simulink model "opt_qvm_bocsh_contr"  (Simulink 4.0)
settings: Solver=ode45  StartTime=0.0  StopTime=10.0  RelTol=1e-3
libraries: simulink_extras x7
settings Model: LastModifiedBy=krangelo  BooleanDataType=on

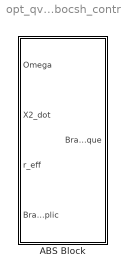
== system opt_qvm_bocsh_contr ==
  ABS Block : Subsystem  SimViewingDevice=off  mask{R1=19000, R2=19000, Bmax=1300, TO=0.006, TC=0.050, Slip=18, Slipmin=17, neg_a=60, pos_a=3, A=10, om_dot_om=3}
      mask prompts: R1 "R1 - Rate of incerase of the  Breake Torque. [Nm/s]"; R2 "R2 - Rate of decerase of the  Breake Torque. [Nm/s]"; Bmax "Bmax - Max. Value of the Brake Torque. [Nm]"; TO "TO - Inlet Valve open time [s]"; TC "TC - Inlet Valve close time [s]"; Slip "Desired slip [%]"; Slipmin "Slipmin - Minimum slip level"; neg_a "-a - Threshold value of the wheel peripheral deceleration [m/s^2]"; pos_a "+a - Threshold value of the wheel peripheral acceleration [m/s^2]"; A "A - Threshold value of the wheel peripheral acceleration [m/s^2]"; om_dot_om "Omdot/Omega -Threshold value of the ratio Om_dot / Om [Hz]"
      settings: Permissions=ReadWrite  RTWFcnNameOpts=Auto  RTWFileNameOpts=Auto

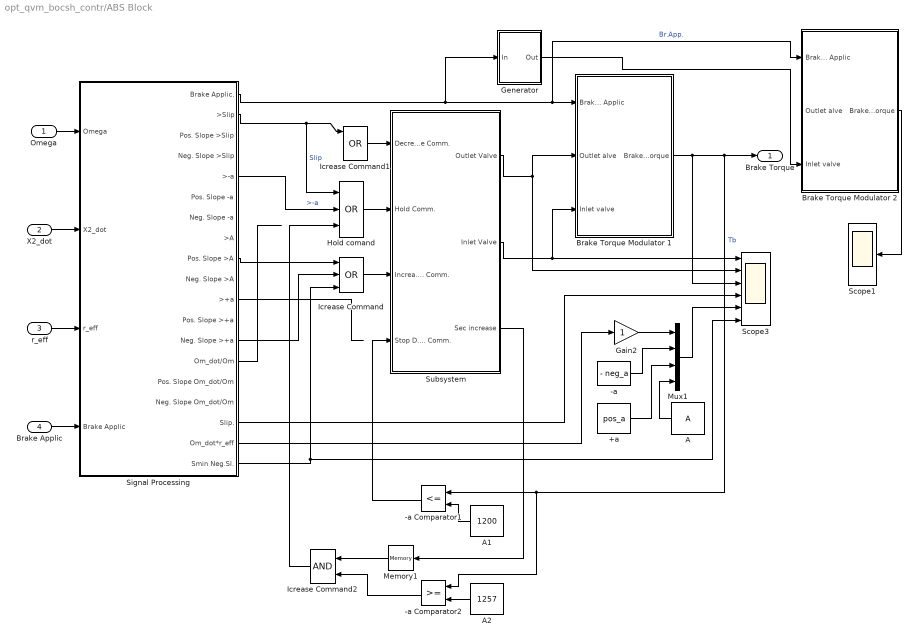
== system opt_qvm_bocsh_contr/ABS Block ==
  Omega : Inport  Port=1  PortDimensions=-1  SampleTime=-1  DataType=auto
      settings: SignalType=auto
  X2_dot : Inport  Port=2  PortDimensions=-1  SampleTime=-1  DataType=auto
      settings: SignalType=auto
  r_eff : Inport  Port=3  PortDimensions=-1  SampleTime=-1  DataType=auto
      settings: SignalType=auto
  Brake Applic : Inport  Port=4  PortDimensions=-1  SampleTime=-1  DataType=auto
      settings: SignalType=auto
  +a : Constant  Value=pos_a
  -a : Constant  Value=- neg_a
  -a Comparator1 : RelationalOperator  Orientation=left  Operator=<=
  -a Comparator2 : RelationalOperator  Orientation=left  Operator=>=
  A : Constant  Orientation=left  Value=A
  A1 : Constant  Orientation=left  Value=1200
  A2 : Constant  Orientation=left  Value=1257
  Brake Torque Modulator 1 : Subsystem  Description=The sysytem holds the Brake Torque at the reached value if no control signal applied  SimViewingDevice=off  mask{Bmax=Bmax, R1=R1, R2=R2}
      mask prompts: Bmax "Bmax - Max. Value of the Brake Torque. [Nm]"; R1 "R1 - Rate of incerase of the  Brake Torque. [Nm/s]"; R2 "R2 - Rate of decerase of the  Brake Torque. [Nm/s]"
      settings: Permissions=ReadWrite  RTWFcnNameOpts=Auto  RTWFileNameOpts=Auto
  Brake Torque Modulator 2 : Subsystem  Description=The sysytem holds the Brake Torque at the reached value if no control signal applied  SimViewingDevice=off  mask{Bmax=Bmax, R1=R1, R2=R2}
      mask prompts: Bmax "Bmax - Max. Value of the Brake Torque. [Nm]"; R1 "R1 - Rate of incerase of the  Brake Torque. [Nm/s]"; R2 "R2 - Rate of decerase of the  Brake Torque. [Nm/s]"
      settings: Permissions=ReadWrite  RTWFcnNameOpts=Auto  RTWFileNameOpts=Auto
  Gain2 : Gain  Gain=1  Multiplication=Element-wise(K.*u)  SaturateOnIntegerOverflow=on
  Generator : Subsystem  SimViewingDevice=off  mask{TO=TO, TC=TC}
      mask prompts: TO "Valve open [s]"; TC "Valve closed [s]"
      settings: Permissions=ReadWrite  RTWFcnNameOpts=Auto  RTWFileNameOpts=Auto
  Hold comand : Logic  Operator=OR  Inputs=3
  Icrease Command : Logic  Operator=OR  Inputs=3
  Icrease Command1 : Logic  Operator=OR  Inputs=3
  Icrease Command2 : Logic  Orientation=left  Operator=AND  Inputs=2
  Memory1 : Memory  Orientation=left  X0=0  InheritSampleTime=off
  Mux1 : Mux  Inputs=4
  Scope1 : Scope
      settings: TimeRange=3  YMin=-1  YMax=1  SaveToWorkspace=off  SaveName=ScopeData5  MaxDataPoints=5000
  Scope3 : Scope  NumInputPorts=6
      settings: TimeRange=3  YMin=0~0~0~-0.025~-90~-5  YMax=1~1~1500~0.225~30~5  SaveToWorkspace=off  SaveName=ScopeData  MaxDataPoints=5000
  Signal Processing : Subsystem  SimViewingDevice=off
      settings: Permissions=ReadWrite  RTWFcnNameOpts=Auto  RTWFileNameOpts=Auto
  Subsystem : Subsystem  SimViewingDevice=off
      settings: Permissions=ReadWrite  RTWFcnNameOpts=Auto  RTWFileNameOpts=Auto
  Brake Torque : Outport  Port=1
  wires:
  Brake Torque Modulator 1/1(Brake Torque) -> Scope3/3, Brake Torque/1, -a Comparator1/1, -a Comparator2/1  "Tb"
  Subsystem/1(Outlet Valve) -> Scope3/2, Brake Torque Modulator 1/2(Outlet alve)
  Subsystem/2(Inlet Valve) -> Scope3/1, Brake Torque Modulator 1/3(Inlet valve)
  Mux1/1 -> Scope3/5
  A/1 -> Mux1/4
  +a/1 -> Mux1/3
  -a/1 -> Mux1/2
  Gain2/1 -> Mux1/1
  Brake Applic/1 -> Signal Processing/4(Brake Applic)
  Omega/1 -> Signal Processing/1(Omega)
  X2_dot/1 -> Signal Processing/2(X2_dot)
  r_eff/1 -> Signal Processing/3(r_eff)
  Signal Processing/5(>-a) -> Hold comand/2  ">-a"
  Signal Processing/1(Brake Applic.) -> Generator/1(In), Brake Torque Modulator 1/1(Brake Applic), Brake Torque Modulator 2/1(Brake Applic)  "Br.App."
  Signal Processing/18(" Om_dot*r_eff") -> Gain2/1
  Signal Processing/17(Slip.) -> Scope3/4
  Signal Processing/11(>+a) -> ?
  Signal Processing/13(Neg. Slope >+a) -> Icrease Command/2
  Signal Processing/14(Om_dot/Om) -> ?
  Signal Processing/9(Pos. Slope >A) -> Icrease Command/1
  Signal Processing/2(>Slip) -> Icrease Command1/1, Hold comand/1  "Slip"
  Hold comand/1 -> Subsystem/2(Hold Comm.)
  Icrease Command/1 -> Subsystem/3(Increase. Comm.)
  Generator/1(Out) -> Brake Torque Modulator 2/3(Inlet valve)
  Brake Torque Modulator 2/1(Brake Torque) -> Scope1/1
  Signal Processing/19(Smin Neg.Sl.) -> Scope3/6, Icrease Command/3
  Icrease Command1/1 -> Subsystem/1(Decrease Comm.)
  A1/1 -> -a Comparator1/2
  -a Comparator1/1 -> Subsystem/4(Stop Dec. Comm.)
  A2/1 -> -a Comparator2/2
  -a Comparator2/1 -> Icrease Command2/2
  Subsystem/3(Sec increase) -> Memory1/1
  Icrease Command2/1 -> Hold comand/3
  Memory1/1 -> Icrease Command2/1

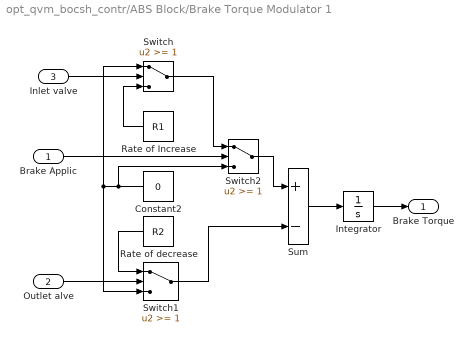
== system opt_qvm_bocsh_contr/ABS Block/Brake Torque Modulator 1 ==
  Brake Applic : Inport  Port=1  PortDimensions=-1  SampleTime=-1  DataType=auto
      settings: SignalType=auto
  Outlet alve : Inport  Port=2  PortDimensions=-1  SampleTime=-1  DataType=auto
      settings: SignalType=auto
  Inlet valve : Inport  Port=3  PortDimensions=-1  SampleTime=-1  DataType=auto
      settings: SignalType=auto
  Constant2 : Constant  Orientation=left  Value=0
  Integrator : Integrator  ExternalReset=none  InitialConditionSource=internal  InitialCondition=0  LimitOutput=on  UpperSaturationLimit=Bmax  LowerSaturationLimit=0  ShowSaturationPort=off  ShowStatePort=off  AbsoluteTolerance=auto
  Rate of Increase : Constant  Orientation=left  Value=R1
  Rate of decrease : Constant  Orientation=left  Value=R2
  Sum : Sum  Inputs=|+-  SaturateOnIntegerOverflow=on
  Switch : Switch  Threshold=1
  Switch1 : Switch  Threshold=1
  Switch2 : Switch  Threshold=1
  Brake Torque : Outport  Port=1
  wires:
  Switch/1 -> Switch2/1
  Brake Applic/1 -> Switch2/2
  Switch2/1 -> Sum/1
  Rate of decrease/1 -> Switch1/1
  Rate of Increase/1 -> Switch/3
  Switch1/1 -> Sum/2
  Integrator/1 -> Brake Torque/1
  Outlet alve/1 -> Switch1/2
  Inlet valve/1 -> Switch/2
  Constant2/1 -> Switch2/3, Switch1/3, Switch/1
  Sum/1 -> Integrator/1

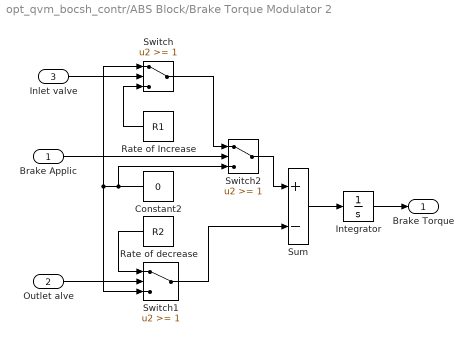
== system opt_qvm_bocsh_contr/ABS Block/Brake Torque Modulator 2 ==
  Brake Applic : Inport  Port=1  PortDimensions=-1  SampleTime=-1  DataType=auto
      settings: SignalType=auto
  Outlet alve : Inport  Port=2  PortDimensions=-1  SampleTime=-1  DataType=auto
      settings: SignalType=auto
  Inlet valve : Inport  Port=3  PortDimensions=-1  SampleTime=-1  DataType=auto
      settings: SignalType=auto
  Constant2 : Constant  Orientation=left  Value=0
  Integrator : Integrator  ExternalReset=none  InitialConditionSource=internal  InitialCondition=0  LimitOutput=on  UpperSaturationLimit=Bmax  LowerSaturationLimit=0  ShowSaturationPort=off  ShowStatePort=off  AbsoluteTolerance=auto
  Rate of Increase : Constant  Orientation=left  Value=R1
  Rate of decrease : Constant  Orientation=left  Value=R2
  Sum : Sum  Inputs=|+-  SaturateOnIntegerOverflow=on
  Switch : Switch  Threshold=1
  Switch1 : Switch  Threshold=1
  Switch2 : Switch  Threshold=1
  Brake Torque : Outport  Port=1
  wires:
  Switch/1 -> Switch2/1
  Brake Applic/1 -> Switch2/2
  Switch2/1 -> Sum/1
  Rate of decrease/1 -> Switch1/1
  Rate of Increase/1 -> Switch/3
  Switch1/1 -> Sum/2
  Integrator/1 -> Brake Torque/1
  Outlet alve/1 -> Switch1/2
  Inlet valve/1 -> Switch/2
  Constant2/1 -> Switch2/3, Switch1/3, Switch/1
  Sum/1 -> Integrator/1

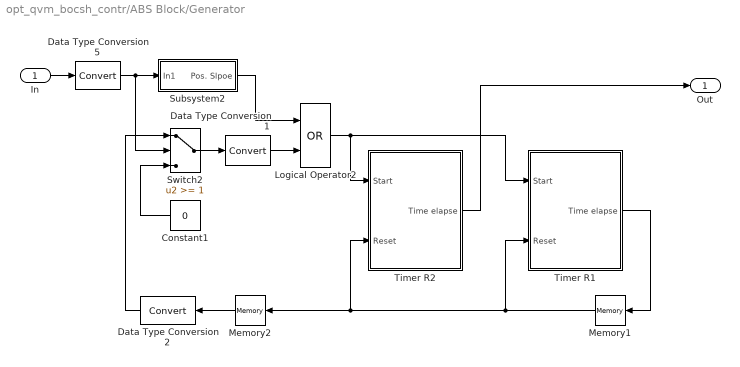
== system opt_qvm_bocsh_contr/ABS Block/Generator ==
  In : Inport  Port=1  PortDimensions=-1  SampleTime=-1  DataType=auto
      settings: SignalType=auto
  Constant1 : Constant  Orientation=left  Value=0
  Data Type Conversion1 : DataTypeConversion  DataType=boolean  SaturateOnIntegerOverflow=on
  Data Type Conversion2 : DataTypeConversion  Orientation=left  DataType=double  SaturateOnIntegerOverflow=on
  Data Type Conversion5 : DataTypeConversion  DataType=boolean  SaturateOnIntegerOverflow=on
  Logical Operator2 : Logic  Operator=OR  Inputs=2
  Memory1 : Memory  Orientation=left  X0=0  InheritSampleTime=off
  Memory2 : Memory  Orientation=left  X0=0  InheritSampleTime=off
  Subsystem2 : Subsystem  SimViewingDevice=off
      settings: Permissions=ReadWrite  RTWFcnNameOpts=Auto  RTWFileNameOpts=Auto
  Switch2 : Switch  Threshold=1
  Timer R1 : Subsystem  SimViewingDevice=off  mask{TC=TC}
      mask prompts: TC "Cycle Time [s]"
      settings: Permissions=ReadWrite  RTWFcnNameOpts=Auto  RTWFileNameOpts=Auto
  Timer R2 : Subsystem  SimViewingDevice=off  mask{TO=TO}
      mask prompts: TO "Open time [s]"
      settings: Permissions=ReadWrite  RTWFcnNameOpts=Auto  RTWFileNameOpts=Auto
  Out : Outport  Port=1
  wires:
  Timer R2/1(Time elapse) -> Out/1
  Data Type Conversion2/1 -> Switch2/1
  Data Type Conversion1/1 -> Logical Operator2/2
  Constant1/1 -> Switch2/3
  Memory2/1 -> Data Type Conversion2/1
  Switch2/1 -> Data Type Conversion1/1
  Memory1/1 -> Memory2/1, Timer R2/2(Reset), Timer R1/2(Reset)
  Data Type Conversion5/1 -> Switch2/2, Subsystem2/1(In1)
  Subsystem2/1(Pos. Slpoe) -> Logical Operator2/1
  In/1 -> Data Type Conversion5/1
  Timer R1/1(Time elapse) -> Memory1/1
  Logical Operator2/1 -> Timer R1/1(Start), Timer R2/1(Start)

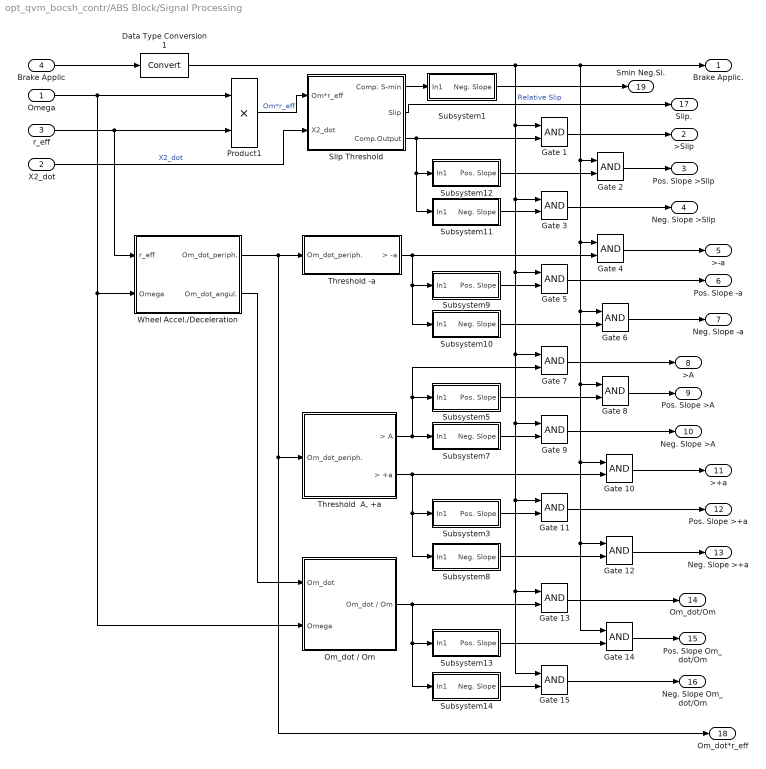
== system opt_qvm_bocsh_contr/ABS Block/Signal Processing ==
  Omega : Inport  Port=1  PortDimensions=-1  SampleTime=-1  DataType=auto
      settings: SignalType=auto
  X2_dot : Inport  Port=2  PortDimensions=-1  SampleTime=-1  DataType=auto
      settings: SignalType=auto
  r_eff : Inport  Port=3  PortDimensions=-1  SampleTime=-1  DataType=auto
      settings: SignalType=auto
  Brake Applic : Inport  Port=4  PortDimensions=-1  SampleTime=-1  DataType=auto
      settings: SignalType=auto
  " Wheel Accel./Deceleration" : Subsystem  SimViewingDevice=off
      settings: Permissions=ReadWrite  RTWFcnNameOpts=Auto  RTWFileNameOpts=Auto
  Data Type Conversion1 : DataTypeConversion  DataType=boolean  SaturateOnIntegerOverflow=on
  Gate {1..15} (15 alike) : Logic  Operator=AND  Inputs=2
  Om_dot / Om : Subsystem  SimViewingDevice=off
      settings: Permissions=ReadWrite  RTWFcnNameOpts=Auto  RTWFileNameOpts=Auto
  Product1 : Product  Inputs=**  Multiplication=Element-wise(.*)  SaturateOnIntegerOverflow=on
  Slip Threshold : Subsystem  SimViewingDevice=off
      settings: Permissions=ReadWrite  RTWFcnNameOpts=Auto  RTWFileNameOpts=Auto
  Subsystem1 : Subsystem  SimViewingDevice=off
      settings: Permissions=ReadWrite  RTWFcnNameOpts=Auto  RTWFileNameOpts=Auto
  Subsystem10 : Subsystem  SimViewingDevice=off
      settings: Permissions=ReadWrite  RTWFcnNameOpts=Auto  RTWFileNameOpts=Auto
  Subsystem11 : Subsystem  SimViewingDevice=off
      settings: Permissions=ReadWrite  RTWFcnNameOpts=Auto  RTWFileNameOpts=Auto
  Subsystem12 : Subsystem  SimViewingDevice=off
      settings: Permissions=ReadWrite  RTWFcnNameOpts=Auto  RTWFileNameOpts=Auto
  Subsystem13 : Subsystem  SimViewingDevice=off
      settings: Permissions=ReadWrite  RTWFcnNameOpts=Auto  RTWFileNameOpts=Auto
  Subsystem14 : Subsystem  SimViewingDevice=off
      settings: Permissions=ReadWrite  RTWFcnNameOpts=Auto  RTWFileNameOpts=Auto
  Subsystem3 : Subsystem  SimViewingDevice=off
      settings: Permissions=ReadWrite  RTWFcnNameOpts=Auto  RTWFileNameOpts=Auto
  Subsystem5 : Subsystem  SimViewingDevice=off
      settings: Permissions=ReadWrite  RTWFcnNameOpts=Auto  RTWFileNameOpts=Auto
  Subsystem7 : Subsystem  SimViewingDevice=off
      settings: Permissions=ReadWrite  RTWFcnNameOpts=Auto  RTWFileNameOpts=Auto
  Subsystem8 : Subsystem  SimViewingDevice=off
      settings: Permissions=ReadWrite  RTWFcnNameOpts=Auto  RTWFileNameOpts=Auto
  Subsystem9 : Subsystem  SimViewingDevice=off
      settings: Permissions=ReadWrite  RTWFcnNameOpts=Auto  RTWFileNameOpts=Auto
  "Threshold  A, +a" : Subsystem  SimViewingDevice=off
      settings: Permissions=ReadWrite  RTWFcnNameOpts=Auto  RTWFileNameOpts=Auto
  Threshold -a : Subsystem  SimViewingDevice=off
      settings: Permissions=ReadWrite  RTWFcnNameOpts=Auto  RTWFileNameOpts=Auto
  Brake Applic. : Outport  Port=1
  >Slip : Outport  Port=2
  Pos. Slope >Slip : Outport  Port=3
  Neg. Slope >Slip : Outport  Port=4
  >-a : Outport  Port=5
  Pos. Slope -a : Outport  Port=6
  Neg. Slope -a : Outport  Port=7
  >A : Outport  Port=8
  Pos. Slope >A : Outport  Port=9
  "Neg. Slope >A " : Outport  Port=10
  >+a : Outport  Port=11
  Pos. Slope >+a : Outport  Port=12
  Neg. Slope >+a : Outport  Port=13
  Om_dot/Om : Outport  Port=14
  Pos. Slope Om_dot/Om : Outport  Port=15
  Neg. Slope Om_dot/Om : Outport  Port=16
  Slip. : Outport  Port=17
  " Om_dot*r_eff" : Outport  Port=18
  Smin Neg.Sl. : Outport  Port=19
  wires:
  Brake Applic/1 -> Data Type Conversion1/1
  Product1/1 -> Slip Threshold/1(Om*r_eff)  "Om*r_eff"
  X2_dot/1 -> Slip Threshold/2(X2_dot)  "X2_dot"
  r_eff/1 -> Product1/2, " Wheel Accel./Deceleration"/1(r_eff)
  Omega/1 -> Om_dot / Om/2(Omega), " Wheel Accel./Deceleration"/2(Omega), Product1/1
  "Threshold  A, +a"/1(" > A") -> Subsystem7/1(In1), Subsystem5/1(In1), Gate 7/2
  "Threshold  A, +a"/2(> +a) -> Subsystem3/1(In1), Subsystem8/1(In1), Gate 10/2
  Subsystem8/1(Neg. Slope) -> Gate 12/2
  Subsystem3/1(Pos. Slope) -> Gate 11/2
  Subsystem7/1(Neg. Slope) -> Gate 9/2
  Subsystem5/1(Pos. Slope) -> Gate 8/2
  Subsystem10/1(Neg. Slope) -> Gate 6/2
  Subsystem9/1(Pos. Slope) -> Gate 5/2
  Threshold -a/1(> -a) -> Subsystem10/1(In1), Subsystem9/1(In1), Gate 4/2
  Subsystem11/1(Neg. Slope) -> Gate 3/2
  Subsystem12/1(Pos. Slope) -> Gate 2/2
  Slip Threshold/3(Comp.Output) -> Subsystem12/1(In1), Subsystem11/1(In1), Gate 1/2
  Om_dot / Om/1(Om_dot / Om) -> Subsystem13/1(In1), Subsystem14/1(In1), Gate 13/2
  Subsystem14/1(Neg. Slope) -> Gate 15/2
  Subsystem13/1(Pos. Slope) -> Gate 14/2
  Data Type Conversion1/1 -> Gate 1/1, Gate 3/1, Gate 5/1, Gate 7/1, Gate 9/1, Gate 11/1, Gate 13/1, Gate 15/1, Brake Applic./1, Gate 2/1, Gate 4/1, Gate 6/1, Gate 8/1, Gate 10/1, Gate 12/1, Gate 14/1
  Gate 1/1 -> >Slip/1
  Gate 2/1 -> Pos. Slope >Slip/1
  Gate 3/1 -> Neg. Slope >Slip/1
  Gate 4/1 -> >-a/1
  Gate 5/1 -> Pos. Slope -a/1
  Gate 6/1 -> Neg. Slope -a/1
  Gate 7/1 -> >A/1
  Gate 8/1 -> Pos. Slope >A/1
  Gate 9/1 -> "Neg. Slope >A "/1
  Gate 10/1 -> >+a/1
  Gate 11/1 -> Pos. Slope >+a/1
  Gate 13/1 -> Om_dot/Om/1
  Gate 14/1 -> Pos. Slope Om_dot/Om/1
  Gate 15/1 -> Neg. Slope Om_dot/Om/1
  " Wheel Accel./Deceleration"/1(Om_dot_periph.) -> " Om_dot*r_eff"/1, "Threshold  A, +a"/1(Om_dot_periph.), Threshold -a/1(Om_dot_periph.)
  Gate 12/1 -> Neg. Slope >+a/1
  Slip Threshold/2(Slip) -> Slip./1  "Relative Slip"
  " Wheel Accel./Deceleration"/2(Om_dot_angul.) -> Om_dot / Om/1(Om_dot)
  Slip Threshold/1(Comp. S-min) -> Subsystem1/1(In1)
  Subsystem1/1(Neg. Slope) -> Smin Neg.Sl./1

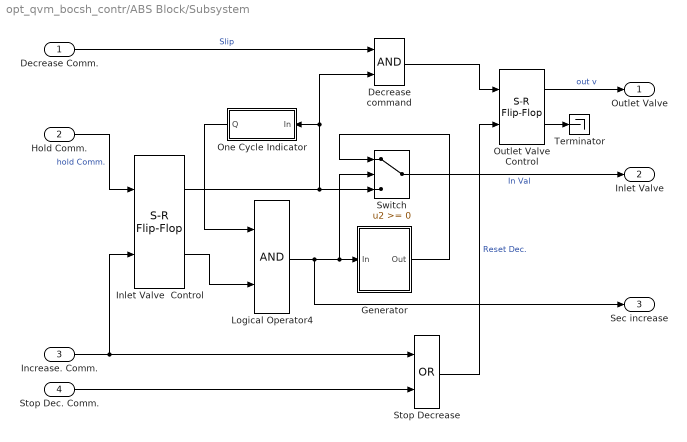
== system opt_qvm_bocsh_contr/ABS Block/Subsystem ==
  Decrease Comm. : Inport  Port=1  PortDimensions=-1  SampleTime=-1  DataType=auto
      settings: SignalType=auto
  Hold Comm. : Inport  Port=2  PortDimensions=-1  SampleTime=-1  DataType=auto
      settings: SignalType=auto
  Increase. Comm. : Inport  Port=3  PortDimensions=-1  SampleTime=-1  DataType=auto
      settings: SignalType=auto
  Stop Dec. Comm. : Inport  Port=4  PortDimensions=-1  SampleTime=-1  DataType=auto
      settings: SignalType=auto
  Decrease command : Logic  Operator=AND  Inputs=2
  Generator : Subsystem  SimViewingDevice=off  mask{TO=TO, TC=TC}
      mask prompts: TO "Valve open [s]"; TC "Valve closed [s]"
      settings: Permissions=ReadWrite  RTWFcnNameOpts=Auto  RTWFileNameOpts=Auto
  Inlet Valve  Control : simulink_extras/Flip Flops/S-R Flip-Flop  initial_condition=0
  Logical Operator4 : Logic  Operator=AND  Inputs=2
  One Cycle Indicator : Subsystem  Orientation=left  SimViewingDevice=off
      settings: Permissions=ReadWrite  RTWFcnNameOpts=Auto  RTWFileNameOpts=Auto
  Outlet Valve Control : simulink_extras/Flip Flops/S-R Flip-Flop  initial_condition=0
  Stop Decrease : Logic  Operator=OR  Inputs=2
  Switch : Switch  Threshold=0
  Terminator : Terminator
  Outlet Valve : Outport  Port=1
  Inlet Valve : Outport  Port=2
  Sec increase : Outport  Port=3
  wires:
  Decrease command/1 -> Outlet Valve Control/1
  Inlet Valve  Control/1 -> Switch/3, Decrease command/2, One Cycle Indicator/1(In)
  Stop Decrease/1 -> Outlet Valve Control/2  "Reset Dec."
  Logical Operator4/1 -> Generator/1(In), Switch/2, Sec increase/1
  Inlet Valve  Control/2 -> Logical Operator4/2
  Generator/1(Out) -> Switch/1
  Decrease Comm./1 -> Decrease command/1  "Slip"
  Outlet Valve Control/1 -> Outlet Valve/1  "out v"
  Hold Comm./1 -> Inlet Valve  Control/1  "hold Comm."
  Switch/1 -> Inlet Valve/1  "In Val"
  Increase. Comm./1 -> Inlet Valve  Control/2, Stop Decrease/1
  Stop Dec. Comm./1 -> Stop Decrease/2
  One Cycle Indicator/1(Q) -> Logical Operator4/1
  Outlet Valve Control/2 -> Terminator/1

== system opt_qvm_bocsh_contr/ABS Block/Generator/Subsystem2 ==
  In1 : Inport  Port=1  PortDimensions=-1  SampleTime=-1  DataType=auto
      settings: SignalType=auto
  Logical Operator2 : Logic  Operator=XOR  Inputs=2
  Logical Operator3 : Logic  Operator=AND  Inputs=2
  Memory : Memory  X0=0  InheritSampleTime=off
  Pos. Slpoe : Outport  Port=1
  wires:
  Logical Operator3/1 -> Pos. Slpoe/1
  In1/1 -> Logical Operator3/1, Memory/1, Logical Operator2/2
  Logical Operator2/1 -> Logical Operator3/2
  Memory/1 -> Logical Operator2/1

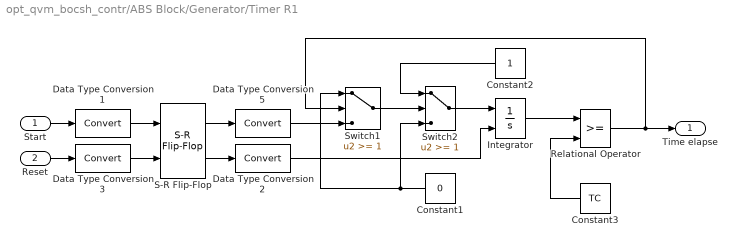
== system opt_qvm_bocsh_contr/ABS Block/Generator/Timer R1 ==
  Start : Inport  Port=1  PortDimensions=-1  SampleTime=-1  DataType=auto
      settings: SignalType=auto
  Reset : Inport  Port=2  PortDimensions=-1  SampleTime=-1  DataType=auto
      settings: SignalType=auto
  Constant1 : Constant  Orientation=left  Value=0
  Constant2 : Constant  Orientation=left  Value=1
  Constant3 : Constant  Orientation=left  Value=TC
  Data Type Conversion1 : DataTypeConversion  DataType=boolean  SaturateOnIntegerOverflow=on
  Data Type Conversion2 : DataTypeConversion  DataType=double  SaturateOnIntegerOverflow=on
  Data Type Conversion3 : DataTypeConversion  DataType=boolean  SaturateOnIntegerOverflow=on
  Data Type Conversion5 : DataTypeConversion  DataType=double  SaturateOnIntegerOverflow=on
  Integrator : Integrator  ExternalReset=level  InitialConditionSource=internal  InitialCondition=0  LimitOutput=off  UpperSaturationLimit=inf  LowerSaturationLimit=-inf  ShowSaturationPort=off  ShowStatePort=off  AbsoluteTolerance=auto
  Relational Operator : RelationalOperator  Operator=>=
  S-R Flip-Flop : simulink_extras/Flip Flops/S-R Flip-Flop  initial_condition=0
  Switch1 : Switch  Threshold=1
  Switch2 : Switch  Threshold=1
  Time elapse : Outport  Port=1
  wires:
  Data Type Conversion5/1 -> Switch1/3
  S-R Flip-Flop/1 -> Data Type Conversion5/1
  Data Type Conversion2/1 -> Integrator/2
  S-R Flip-Flop/2 -> Data Type Conversion2/1
  Start/1 -> Data Type Conversion1/1
  Data Type Conversion1/1 -> S-R Flip-Flop/1
  Reset/1 -> Data Type Conversion3/1
  Data Type Conversion3/1 -> S-R Flip-Flop/2
  Switch2/1 -> Integrator/1
  Constant3/1 -> Relational Operator/2
  Constant1/1 -> Switch1/1, Switch2/3
  Integrator/1 -> Relational Operator/1
  Relational Operator/1 -> Switch1/2, Time elapse/1
  Switch1/1 -> Switch2/2
  Constant2/1 -> Switch2/1

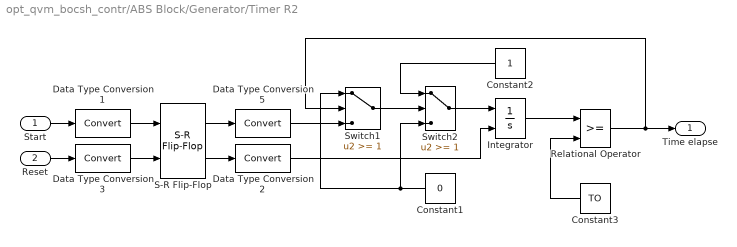
== system opt_qvm_bocsh_contr/ABS Block/Generator/Timer R2 ==
  Start : Inport  Port=1  PortDimensions=-1  SampleTime=-1  DataType=auto
      settings: SignalType=auto
  Reset : Inport  Port=2  PortDimensions=-1  SampleTime=-1  DataType=auto
      settings: SignalType=auto
  Constant1 : Constant  Orientation=left  Value=0
  Constant2 : Constant  Orientation=left  Value=1
  Constant3 : Constant  Orientation=left  Value=TO
  Data Type Conversion1 : DataTypeConversion  DataType=boolean  SaturateOnIntegerOverflow=on
  Data Type Conversion2 : DataTypeConversion  DataType=double  SaturateOnIntegerOverflow=on
  Data Type Conversion3 : DataTypeConversion  DataType=boolean  SaturateOnIntegerOverflow=on
  Data Type Conversion5 : DataTypeConversion  DataType=double  SaturateOnIntegerOverflow=on
  Integrator : Integrator  ExternalReset=level  InitialConditionSource=internal  InitialCondition=0  LimitOutput=off  UpperSaturationLimit=inf  LowerSaturationLimit=-inf  ShowSaturationPort=off  ShowStatePort=off  AbsoluteTolerance=auto
  Relational Operator : RelationalOperator  Operator=>=
  S-R Flip-Flop : simulink_extras/Flip Flops/S-R Flip-Flop  initial_condition=0
  Switch1 : Switch  Threshold=1
  Switch2 : Switch  Threshold=1
  Time elapse : Outport  Port=1
  wires:
  Data Type Conversion5/1 -> Switch1/3
  S-R Flip-Flop/1 -> Data Type Conversion5/1
  Data Type Conversion2/1 -> Integrator/2
  S-R Flip-Flop/2 -> Data Type Conversion2/1
  Start/1 -> Data Type Conversion1/1
  Data Type Conversion1/1 -> S-R Flip-Flop/1
  Reset/1 -> Data Type Conversion3/1
  Data Type Conversion3/1 -> S-R Flip-Flop/2
  Switch2/1 -> Integrator/1
  Constant3/1 -> Relational Operator/2
  Constant1/1 -> Switch1/1, Switch2/3
  Integrator/1 -> Relational Operator/1
  Relational Operator/1 -> Switch1/2, Time elapse/1
  Switch1/1 -> Switch2/2
  Constant2/1 -> Switch2/1

== system opt_qvm_bocsh_contr/ABS Block/Signal Processing/ Wheel Accel./Deceleration ==
  r_eff : Inport  Port=1  PortDimensions=-1  SampleTime=-1  DataType=auto
      settings: SignalType=auto
  Omega : Inport  Port=2  PortDimensions=-1  SampleTime=-1  DataType=auto
      settings: SignalType=auto
  Derivative : Derivative
  Low-pass filter : TransferFcn  Numerator=[1.15]  Denominator=[0.0105 1]  AbsoluteTolerance=auto  Realization=auto
  Product2 : Product  Inputs=**  Multiplication=Element-wise(.*)  SaturateOnIntegerOverflow=on
  To Workspace1 : ToWorkspace  VariableName=om_dot_per  SampleTime=0  SaveFormat=Array
      settings: MaxDataPoints=10000
  To Workspace3 : ToWorkspace  VariableName=om_dotcont  SampleTime=0  SaveFormat=Array
      settings: MaxDataPoints=10000
  Om_dot_periph. : Outport  Port=1
  Om_dot_angul. : Outport  Port=2
  wires:
  Low-pass filter/1 -> Product2/2, Om_dot_angul./1  "om_dot"
  Derivative/1 -> Low-pass filter/1, To Workspace3/1  "dot"
  r_eff/1 -> Product2/1
  Omega/1 -> Derivative/1
  Product2/1 -> Om_dot_periph./1, To Workspace1/1

== system opt_qvm_bocsh_contr/ABS Block/Signal Processing/Om_dot / Om ==
  Om_dot : Inport  Port=1  PortDimensions=-1  SampleTime=-1  DataType=auto
      settings: SignalType=auto
  Omega : Inport  Port=2  PortDimensions=-1  SampleTime=-1  DataType=auto
      settings: SignalType=auto
  Gain2 : Gain  Gain=-1  Multiplication=Element-wise(K.*u)  SaturateOnIntegerOverflow=on
  Product : Product  Inputs=*/  Multiplication=Element-wise(.*)  SaturateOnIntegerOverflow=on
  Relational Operator1 : RelationalOperator  Operator=>
  Threshold Value : Constant  Orientation=left  Value=om_dot_om
  To Workspace2 : ToWorkspace  VariableName=om_dotf_om  SampleTime=0  SaveFormat=Array
      settings: MaxDataPoints=10000
  Om_dot / Om : Outport  Port=1
  wires:
  Threshold Value/1 -> Relational Operator1/2
  Product/1 -> Relational Operator1/1, To Workspace2/1
  Gain2/1 -> Product/1
  Om_dot/1 -> Gain2/1
  Relational Operator1/1 -> Om_dot / Om/1
  Omega/1 -> Product/2

== system opt_qvm_bocsh_contr/ABS Block/Signal Processing/Slip Threshold ==
  Om*r_eff : Inport  Port=1  PortDimensions=-1  SampleTime=-1  DataType=auto
      settings: SignalType=auto
  X2_dot : Inport  Port=2  PortDimensions=-1  SampleTime=-1  DataType=auto
      settings: SignalType=auto
  " Slip Computation" : Fcn  Expr=1.0 - u(1)/u(2)
  Mux : Mux  Inputs=2
  Slip Comparator : RelationalOperator  Operator=>
  Slip Comparator1 : RelationalOperator  Operator=>
  Slip set-poit : Constant  Orientation=left  Value=0.01*Slip
  Slip set-poit1 : Constant  Orientation=left  Value=0.01*Slipmin
  To Workspace18 : ToWorkspace  VariableName=slip_est  SampleTime=0  SaveFormat=Array
      settings: MaxDataPoints=10000
  Comp. S-min : Outport  Port=1
  Slip : Outport  Port=2
  Comp.Output : Outport  Port=3
  wires:
  Slip set-poit/1 -> Slip Comparator/2
  Mux/1 -> " Slip Computation"/1  "Vehicle-Wheel Vel."
  " Slip Computation"/1 -> To Workspace18/1, Slip Comparator/1, Slip/1, Slip Comparator1/1
  Om*r_eff/1 -> Mux/1
  Slip Comparator/1 -> Comp.Output/1  "Slip exceed"
  X2_dot/1 -> Mux/2
  Slip set-poit1/1 -> Slip Comparator1/2
  Slip Comparator1/1 -> Comp. S-min/1  "Slip exceed"

== system opt_qvm_bocsh_contr/ABS Block/Signal Processing/Subsystem1 ==
  In1 : Inport  Port=1  PortDimensions=-1  SampleTime=-1  DataType=auto
      settings: SignalType=auto
  Logical Operator2 : Logic  Operator=XOR  Inputs=2
  Logical Operator3 : Logic  Operator=AND  Inputs=2
  Memory : Memory  X0=0  InheritSampleTime=off
  Neg. Slope : Outport  Port=1
  wires:
  Logical Operator3/1 -> Neg. Slope/1
  In1/1 -> Logical Operator2/2, Memory/1
  Logical Operator2/1 -> Logical Operator3/2
  Memory/1 -> Logical Operator3/1, Logical Operator2/1

== system opt_qvm_bocsh_contr/ABS Block/Signal Processing/Subsystem10 ==
  In1 : Inport  Port=1  PortDimensions=-1  SampleTime=-1  DataType=auto
      settings: SignalType=auto
  Logical Operator2 : Logic  Operator=XOR  Inputs=2
  Logical Operator3 : Logic  Operator=AND  Inputs=2
  Memory : Memory  X0=0  InheritSampleTime=off
  Neg. Slope : Outport  Port=1
  wires:
  Logical Operator3/1 -> Neg. Slope/1
  In1/1 -> Logical Operator2/2, Memory/1
  Logical Operator2/1 -> Logical Operator3/2
  Memory/1 -> Logical Operator3/1, Logical Operator2/1

== system opt_qvm_bocsh_contr/ABS Block/Signal Processing/Subsystem11 ==
  In1 : Inport  Port=1  PortDimensions=-1  SampleTime=-1  DataType=auto
      settings: SignalType=auto
  Logical Operator2 : Logic  Operator=XOR  Inputs=2
  Logical Operator3 : Logic  Operator=AND  Inputs=2
  Memory : Memory  X0=0  InheritSampleTime=off
  Neg. Slope : Outport  Port=1
  wires:
  Logical Operator3/1 -> Neg. Slope/1
  In1/1 -> Logical Operator2/2, Memory/1
  Logical Operator2/1 -> Logical Operator3/2
  Memory/1 -> Logical Operator3/1, Logical Operator2/1

== system opt_qvm_bocsh_contr/ABS Block/Signal Processing/Subsystem12 ==
  In1 : Inport  Port=1  PortDimensions=-1  SampleTime=-1  DataType=auto
      settings: SignalType=auto
  Logical Operator2 : Logic  Operator=XOR  Inputs=2
  Logical Operator3 : Logic  Operator=AND  Inputs=2
  Memory : Memory  X0=0  InheritSampleTime=off
  Pos. Slope : Outport  Port=1
  wires:
  Logical Operator3/1 -> Pos. Slope/1
  In1/1 -> Logical Operator2/2, Memory/1, Logical Operator3/1
  Logical Operator2/1 -> Logical Operator3/2
  Memory/1 -> Logical Operator2/1

== system opt_qvm_bocsh_contr/ABS Block/Signal Processing/Subsystem13 ==
  In1 : Inport  Port=1  PortDimensions=-1  SampleTime=-1  DataType=auto
      settings: SignalType=auto
  Logical Operator2 : Logic  Operator=XOR  Inputs=2
  Logical Operator3 : Logic  Operator=AND  Inputs=2
  Memory : Memory  X0=0  InheritSampleTime=off
  Pos. Slope : Outport  Port=1
  wires:
  Logical Operator3/1 -> Pos. Slope/1
  In1/1 -> Logical Operator2/2, Memory/1, Logical Operator3/1
  Logical Operator2/1 -> Logical Operator3/2
  Memory/1 -> Logical Operator2/1

== system opt_qvm_bocsh_contr/ABS Block/Signal Processing/Subsystem14 ==
  In1 : Inport  Port=1  PortDimensions=-1  SampleTime=-1  DataType=auto
      settings: SignalType=auto
  Logical Operator2 : Logic  Operator=XOR  Inputs=2
  Logical Operator3 : Logic  Operator=AND  Inputs=2
  Memory : Memory  X0=0  InheritSampleTime=off
  Neg. Slope : Outport  Port=1
  wires:
  Logical Operator3/1 -> Neg. Slope/1
  In1/1 -> Logical Operator2/2, Memory/1
  Logical Operator2/1 -> Logical Operator3/2
  Memory/1 -> Logical Operator3/1, Logical Operator2/1

== system opt_qvm_bocsh_contr/ABS Block/Signal Processing/Subsystem3 ==
  In1 : Inport  Port=1  PortDimensions=-1  SampleTime=-1  DataType=auto
      settings: SignalType=auto
  Logical Operator2 : Logic  Operator=XOR  Inputs=2
  Logical Operator3 : Logic  Operator=AND  Inputs=2
  Memory : Memory  X0=0  InheritSampleTime=off
  Pos. Slope : Outport  Port=1
  wires:
  Logical Operator3/1 -> Pos. Slope/1
  In1/1 -> Logical Operator2/2, Memory/1, Logical Operator3/1
  Logical Operator2/1 -> Logical Operator3/2
  Memory/1 -> Logical Operator2/1

== system opt_qvm_bocsh_contr/ABS Block/Signal Processing/Subsystem5 ==
  In1 : Inport  Port=1  PortDimensions=-1  SampleTime=-1  DataType=auto
      settings: SignalType=auto
  Logical Operator2 : Logic  Operator=XOR  Inputs=2
  Logical Operator3 : Logic  Operator=AND  Inputs=2
  Memory : Memory  X0=0  InheritSampleTime=off
  Pos. Slope : Outport  Port=1
  wires:
  Logical Operator3/1 -> Pos. Slope/1
  In1/1 -> Logical Operator2/2, Memory/1, Logical Operator3/1
  Logical Operator2/1 -> Logical Operator3/2
  Memory/1 -> Logical Operator2/1

== system opt_qvm_bocsh_contr/ABS Block/Signal Processing/Subsystem7 ==
  In1 : Inport  Port=1  PortDimensions=-1  SampleTime=-1  DataType=auto
      settings: SignalType=auto
  Logical Operator2 : Logic  Operator=XOR  Inputs=2
  Logical Operator3 : Logic  Operator=AND  Inputs=2
  Memory : Memory  X0=0  InheritSampleTime=off
  Neg. Slope : Outport  Port=1
  wires:
  Logical Operator3/1 -> Neg. Slope/1
  In1/1 -> Logical Operator2/2, Memory/1
  Logical Operator2/1 -> Logical Operator3/2
  Memory/1 -> Logical Operator3/1, Logical Operator2/1

== system opt_qvm_bocsh_contr/ABS Block/Signal Processing/Subsystem8 ==
  In1 : Inport  Port=1  PortDimensions=-1  SampleTime=-1  DataType=auto
      settings: SignalType=auto
  Logical Operator2 : Logic  Operator=XOR  Inputs=2
  Logical Operator3 : Logic  Operator=AND  Inputs=2
  Memory : Memory  X0=0  InheritSampleTime=off
  Neg. Slope : Outport  Port=1
  wires:
  Logical Operator3/1 -> Neg. Slope/1
  In1/1 -> Logical Operator2/2, Memory/1
  Logical Operator2/1 -> Logical Operator3/2
  Memory/1 -> Logical Operator3/1, Logical Operator2/1

== system opt_qvm_bocsh_contr/ABS Block/Signal Processing/Subsystem9 ==
  In1 : Inport  Port=1  PortDimensions=-1  SampleTime=-1  DataType=auto
      settings: SignalType=auto
  Logical Operator2 : Logic  Operator=XOR  Inputs=2
  Logical Operator3 : Logic  Operator=AND  Inputs=2
  Memory : Memory  X0=0  InheritSampleTime=off
  Pos. Slope : Outport  Port=1
  wires:
  Logical Operator3/1 -> Pos. Slope/1
  In1/1 -> Logical Operator2/2, Memory/1, Logical Operator3/1
  Logical Operator2/1 -> Logical Operator3/2
  Memory/1 -> Logical Operator2/1

== system opt_qvm_bocsh_contr/ABS Block/Signal Processing/Threshold  A, +a ==
  Om_dot_periph. : Inport  Port=1  PortDimensions=-1  SampleTime=-1  DataType=auto
      settings: SignalType=auto
  +a Comparator1 : RelationalOperator  Operator=>
  +a positive acc. : Constant  Orientation=left  Value=pos_a
  A Comparator : RelationalOperator  Operator=>
  A positive acc. : Constant  Orientation=left  Value=A
  " > A" : Outport  Port=1
  > +a : Outport  Port=2
  wires:
  +a Comparator1/1 -> > +a/1
  +a positive acc./1 -> +a Comparator1/2
  A Comparator/1 -> " > A"/1
  A positive acc./1 -> A Comparator/2
  Om_dot_periph./1 -> A Comparator/1, +a Comparator1/1

== system opt_qvm_bocsh_contr/ABS Block/Signal Processing/Threshold -a ==
  Om_dot_periph. : Inport  Port=1  PortDimensions=-1  SampleTime=-1  DataType=auto
      settings: SignalType=auto
  -a Comparator1 : RelationalOperator  Operator=>=
  -a negative acc. : Constant  Orientation=left  Value=neg_a
  Gain2 : Gain  Gain=-1  Multiplication=Element-wise(K.*u)  SaturateOnIntegerOverflow=on
  > -a : Outport  Port=1
  wires:
  Gain2/1 -> -a Comparator1/1
  -a Comparator1/1 -> > -a/1
  -a negative acc./1 -> -a Comparator1/2
  Om_dot_periph./1 -> Gain2/1

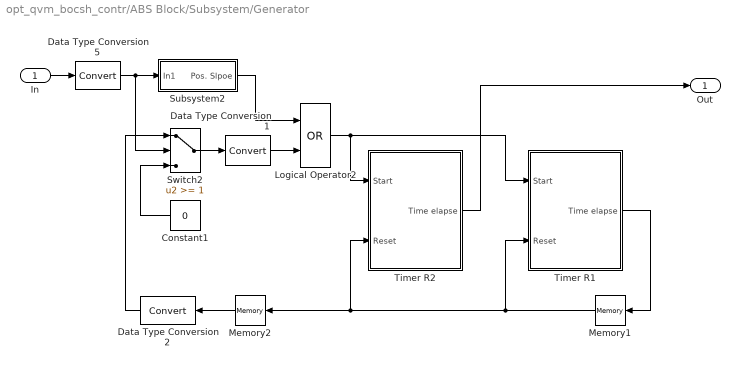
== system opt_qvm_bocsh_contr/ABS Block/Subsystem/Generator ==
  In : Inport  Port=1  PortDimensions=-1  SampleTime=-1  DataType=auto
      settings: SignalType=auto
  Constant1 : Constant  Orientation=left  Value=0
  Data Type Conversion1 : DataTypeConversion  DataType=boolean  SaturateOnIntegerOverflow=on
  Data Type Conversion2 : DataTypeConversion  Orientation=left  DataType=double  SaturateOnIntegerOverflow=on
  Data Type Conversion5 : DataTypeConversion  DataType=boolean  SaturateOnIntegerOverflow=on
  Logical Operator2 : Logic  Operator=OR  Inputs=2
  Memory1 : Memory  Orientation=left  X0=0  InheritSampleTime=off
  Memory2 : Memory  Orientation=left  X0=0  InheritSampleTime=off
  Subsystem2 : Subsystem  SimViewingDevice=off
      settings: Permissions=ReadWrite  RTWFcnNameOpts=Auto  RTWFileNameOpts=Auto
  Switch2 : Switch  Threshold=1
  Timer R1 : Subsystem  SimViewingDevice=off  mask{TC=TC}
      mask prompts: TC "Cycle Time [s]"
      settings: Permissions=ReadWrite  RTWFcnNameOpts=Auto  RTWFileNameOpts=Auto
  Timer R2 : Subsystem  SimViewingDevice=off  mask{TO=TO}
      mask prompts: TO "Open time [s]"
      settings: Permissions=ReadWrite  RTWFcnNameOpts=Auto  RTWFileNameOpts=Auto
  Out : Outport  Port=1
  wires:
  Timer R2/1(Time elapse) -> Out/1
  Data Type Conversion2/1 -> Switch2/1
  Data Type Conversion1/1 -> Logical Operator2/2
  Constant1/1 -> Switch2/3
  Memory2/1 -> Data Type Conversion2/1
  Switch2/1 -> Data Type Conversion1/1
  Memory1/1 -> Memory2/1, Timer R2/2(Reset), Timer R1/2(Reset)
  Data Type Conversion5/1 -> Switch2/2, Subsystem2/1(In1)
  Subsystem2/1(Pos. Slpoe) -> Logical Operator2/1
  In/1 -> Data Type Conversion5/1
  Timer R1/1(Time elapse) -> Memory1/1
  Logical Operator2/1 -> Timer R1/1(Start), Timer R2/1(Start)

== system opt_qvm_bocsh_contr/ABS Block/Subsystem/One Cycle Indicator ==
  In : Inport  Port=1  PortDimensions=-1  SampleTime=-1  DataType=auto
      settings: SignalType=auto
  Logical Operator3 : Logic  Operator=OR  Inputs=2
  Memory : Memory  X0=0  InheritSampleTime=off
  S-R Flip-Flop : simulink_extras/Flip Flops/S-R Flip-Flop  Orientation=left  initial_condition=0
  Terminator : Terminator
  Q : Outport  Port=1
  wires:
  S-R Flip-Flop/2 -> Terminator/1
  In/1 -> Logical Operator3/2
  S-R Flip-Flop/1 -> Memory/1
  Memory/1 -> Q/1, Logical Operator3/1
  Logical Operator3/1 -> S-R Flip-Flop/1

== system opt_qvm_bocsh_contr/ABS Block/Subsystem/Generator/Subsystem2 ==
  In1 : Inport  Port=1  PortDimensions=-1  SampleTime=-1  DataType=auto
      settings: SignalType=auto
  Logical Operator2 : Logic  Operator=XOR  Inputs=2
  Logical Operator3 : Logic  Operator=AND  Inputs=2
  Memory : Memory  X0=0  InheritSampleTime=off
  Pos. Slpoe : Outport  Port=1
  wires:
  Logical Operator3/1 -> Pos. Slpoe/1
  In1/1 -> Logical Operator3/1, Memory/1, Logical Operator2/2
  Logical Operator2/1 -> Logical Operator3/2
  Memory/1 -> Logical Operator2/1

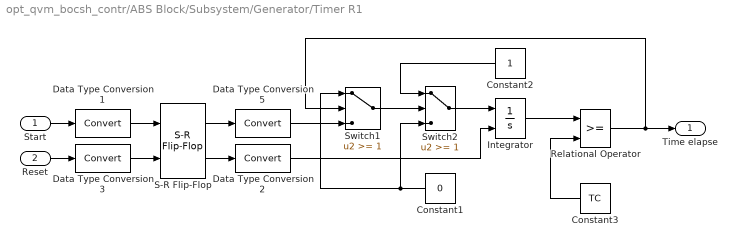
== system opt_qvm_bocsh_contr/ABS Block/Subsystem/Generator/Timer R1 ==
  Start : Inport  Port=1  PortDimensions=-1  SampleTime=-1  DataType=auto
      settings: SignalType=auto
  Reset : Inport  Port=2  PortDimensions=-1  SampleTime=-1  DataType=auto
      settings: SignalType=auto
  Constant1 : Constant  Orientation=left  Value=0
  Constant2 : Constant  Orientation=left  Value=1
  Constant3 : Constant  Orientation=left  Value=TC
  Data Type Conversion1 : DataTypeConversion  DataType=boolean  SaturateOnIntegerOverflow=on
  Data Type Conversion2 : DataTypeConversion  DataType=double  SaturateOnIntegerOverflow=on
  Data Type Conversion3 : DataTypeConversion  DataType=boolean  SaturateOnIntegerOverflow=on
  Data Type Conversion5 : DataTypeConversion  DataType=double  SaturateOnIntegerOverflow=on
  Integrator : Integrator  ExternalReset=level  InitialConditionSource=internal  InitialCondition=0  LimitOutput=off  UpperSaturationLimit=inf  LowerSaturationLimit=-inf  ShowSaturationPort=off  ShowStatePort=off  AbsoluteTolerance=auto
  Relational Operator : RelationalOperator  Operator=>=
  S-R Flip-Flop : simulink_extras/Flip Flops/S-R Flip-Flop  initial_condition=0
  Switch1 : Switch  Threshold=1
  Switch2 : Switch  Threshold=1
  Time elapse : Outport  Port=1
  wires:
  Data Type Conversion5/1 -> Switch1/3
  S-R Flip-Flop/1 -> Data Type Conversion5/1
  Data Type Conversion2/1 -> Integrator/2
  S-R Flip-Flop/2 -> Data Type Conversion2/1
  Start/1 -> Data Type Conversion1/1
  Data Type Conversion1/1 -> S-R Flip-Flop/1
  Reset/1 -> Data Type Conversion3/1
  Data Type Conversion3/1 -> S-R Flip-Flop/2
  Switch2/1 -> Integrator/1
  Constant3/1 -> Relational Operator/2
  Constant1/1 -> Switch1/1, Switch2/3
  Integrator/1 -> Relational Operator/1
  Relational Operator/1 -> Switch1/2, Time elapse/1
  Switch1/1 -> Switch2/2
  Constant2/1 -> Switch2/1

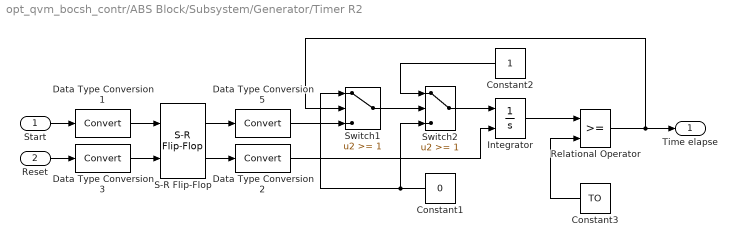
== system opt_qvm_bocsh_contr/ABS Block/Subsystem/Generator/Timer R2 ==
  Start : Inport  Port=1  PortDimensions=-1  SampleTime=-1  DataType=auto
      settings: SignalType=auto
  Reset : Inport  Port=2  PortDimensions=-1  SampleTime=-1  DataType=auto
      settings: SignalType=auto
  Constant1 : Constant  Orientation=left  Value=0
  Constant2 : Constant  Orientation=left  Value=1
  Constant3 : Constant  Orientation=left  Value=TO
  Data Type Conversion1 : DataTypeConversion  DataType=boolean  SaturateOnIntegerOverflow=on
  Data Type Conversion2 : DataTypeConversion  DataType=double  SaturateOnIntegerOverflow=on
  Data Type Conversion3 : DataTypeConversion  DataType=boolean  SaturateOnIntegerOverflow=on
  Data Type Conversion5 : DataTypeConversion  DataType=double  SaturateOnIntegerOverflow=on
  Integrator : Integrator  ExternalReset=level  InitialConditionSource=internal  InitialCondition=0  LimitOutput=off  UpperSaturationLimit=inf  LowerSaturationLimit=-inf  ShowSaturationPort=off  ShowStatePort=off  AbsoluteTolerance=auto
  Relational Operator : RelationalOperator  Operator=>=
  S-R Flip-Flop : simulink_extras/Flip Flops/S-R Flip-Flop  initial_condition=0
  Switch1 : Switch  Threshold=1
  Switch2 : Switch  Threshold=1
  Time elapse : Outport  Port=1
  wires:
  Data Type Conversion5/1 -> Switch1/3
  S-R Flip-Flop/1 -> Data Type Conversion5/1
  Data Type Conversion2/1 -> Integrator/2
  S-R Flip-Flop/2 -> Data Type Conversion2/1
  Start/1 -> Data Type Conversion1/1
  Data Type Conversion1/1 -> S-R Flip-Flop/1
  Reset/1 -> Data Type Conversion3/1
  Data Type Conversion3/1 -> S-R Flip-Flop/2
  Switch2/1 -> Integrator/1
  Constant3/1 -> Relational Operator/2
  Constant1/1 -> Switch1/1, Switch2/3
  Integrator/1 -> Relational Operator/1
  Relational Operator/1 -> Switch1/2, Time elapse/1
  Switch1/1 -> Switch2/2
  Constant2/1 -> Switch2/1
